simulink subsystem "robot_model_7dof_ref_subsys"  (R2022b)
settings: Solver=VariableStepAuto  StartTime=0.0  StopTime=10.0  RelTol=1e-3
undefined symbols (not defined in the file): param_robot, param_traj, q_0
settings Model: Creator=emu  LastModifiedBy=rslstudent
settings OptimizationCC: ReuseModelBlockBuffer=on

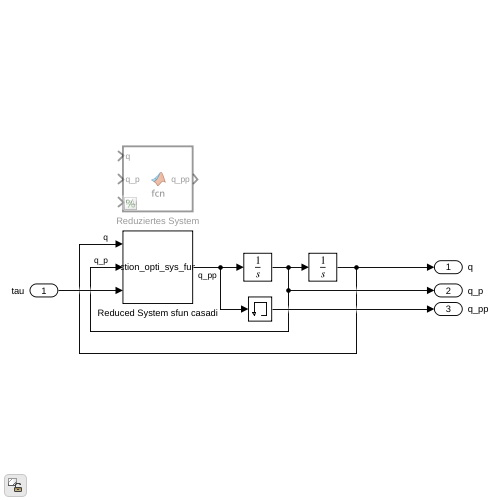
[thumbnail: Simulink's stored preview of the top-level diagram]
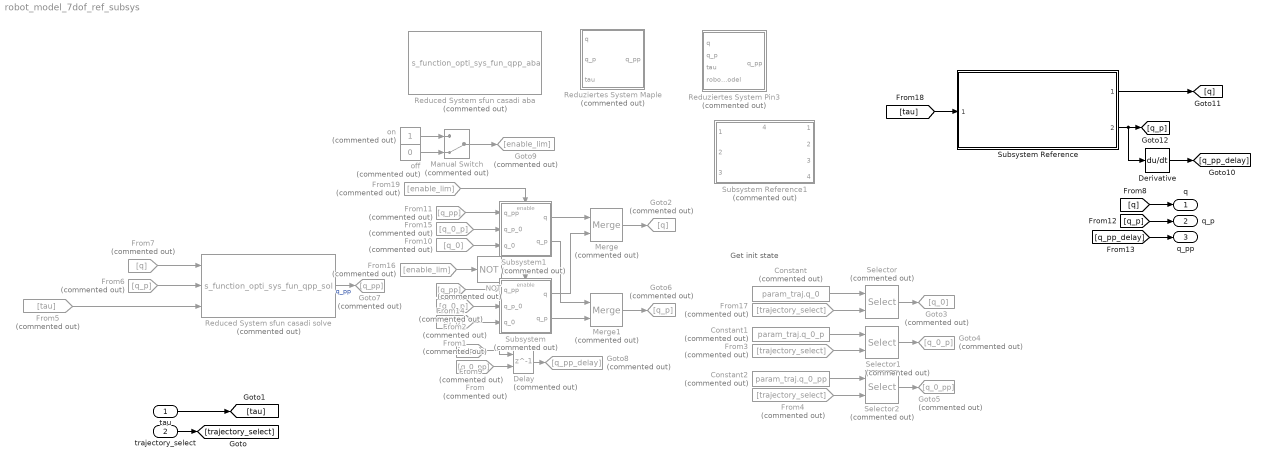
== system robot_model_7dof_ref_subsys ==
  note: Get init state
  tau : Inport
  trajectory_select : Inport  Port=2
  Constant : Constant  Commented=on  Value=param_traj.q_0
  Constant1 : Constant  Commented=on  Value=param_traj.q_0_p
  Constant2 : Constant  Commented=on  Value=param_traj.q_0_pp
  Delay : Delay  Commented=on  DelayLength=1  InitialConditionSource=Input port
      settings: InputPortMap=u0,p4
  Derivative : Derivative
  From : From  Commented=on  GotoTag=q_0_pp
  From1 : From  Commented=on  GotoTag=q_0
  From10 : From  Commented=on  GotoTag=q_0
  From11 : From  Commented=on  GotoTag=q_pp
  From14 : From  Commented=on  GotoTag=q_pp
  From15 : From  Commented=on  GotoTag=q_0_p
  From16 : From  Commented=on  GotoTag=enable_lim
  From17 : From  Commented=on  GotoTag=trajectory_select
  From19 : From  Commented=on  GotoTag=enable_lim
  From2 : From  Commented=on  GotoTag=q_0_p
  From3 : From  Commented=on  GotoTag=trajectory_select
  From4 : From  Commented=on  GotoTag=trajectory_select
  From5 : From  Commented=on  GotoTag=tau
  From6 : From  Commented=on  GotoTag=q_p
  From7 : From  Commented=on  GotoTag=q
  From9 : From  Commented=on  GotoTag=q_pp
  Goto2 : Goto  Commented=on  GotoTag=q
  Goto3 : Goto  Commented=on  GotoTag=q_0
  Goto4 : Goto  Commented=on  GotoTag=q_0_p
  Goto5 : Goto  Commented=on  GotoTag=q_0_pp
  Goto6 : Goto  Commented=on  GotoTag=q_p
  Goto7 : Goto  Commented=on  GotoTag=q_pp
  Goto8 : Goto  Commented=on  GotoTag=q_pp_delay
  Goto9 : Goto  Commented=on  GotoTag=enable_lim
  Manual Switch : ManualSwitch  Commented=on  CurrentSetting=0
  Merge : Merge  Commented=on
  Merge1 : Merge  Commented=on
  NOT : Logic  Commented=on  Operator=NOT  IconShape=distinctive  AllPortsSameDT=off  OutDataTypeStr=boolean
  Reduced System sfun casadi aba : S-Function  Commented=on  FunctionName=s_function_opti_sys_fun_qpp_aba  SFunctionModules='sys_fun_qpp_aba'  SFunctionDeploymentMode=off  EnableBusSupport=off
  Reduced System sfun casadi solve : S-Function  Commented=on  FunctionName=s_function_opti_sys_fun_qpp_sol  SFunctionModules='sys_fun_qpp_sol'  SFunctionDeploymentMode=off  EnableBusSupport=off
  Reduziertes System Maple : MATLAB Function  Commented=on
  Reduziertes System Pin3 : MATLAB Function  Commented=on
  Selector : Selector  Commented=on  NumberOfDimensions=2  InputPortWidth=3  IndexOptions=Index vector (dialog),Index vector (port)  Indices=1:param_robot.n_DOF,1  OutputSizes=1,1
  Selector1 : Selector  Commented=on  NumberOfDimensions=2  InputPortWidth=3  IndexOptions=Index vector (dialog),Index vector (port)  Indices=1:param_robot.n_DOF,1  OutputSizes=1,1
  Selector2 : Selector  Commented=on  NumberOfDimensions=2  InputPortWidth=3  IndexOptions=Index vector (dialog),Index vector (port)  Indices=1:param_robot.n_DOF,1  OutputSizes=1,1
  Subsystem : Subsystem  Commented=on
  Subsystem Reference : Subsystem  ReferencedSubsystem=franka_fr3_no_hand_simscape_model_refsys
  Subsystem Reference1 : Subsystem  Commented=on  ReferencedSubsystem=limit_joint_coordinates_ref_subsys
      settings: PortSchema="{\"entries\":[{\"content\":{\"sides\":[{\"content\":{\"connectorIds\":[\"In1\",\"In2\",\"In3\"]},\"type\":\"ConnectorPlacement.EquallySpacedRectSide\",\"uuid\":\"c83c87ef-f061-4ba1-866a-9dee58807a3f\"},{\"content\":{\"connectorIds\":[\"Out1\",\"Out2\",\"Out3\",\"Out4\"],\"side\":\"RIGHT\"},\"type\":\"ConnectorPlacement.EquallySpacedRectSide\",\"uuid\":\"387cc6c9-8217-4e2c-af30-f5a1ca09c27e\"},{\"content\":{\"connectorIds\":[\"In4\"],\"side\":\"TOP\"},\"type\":\"ConnectorPlacement.EquallySpacedRectSide\",\"uuid\":\"e929a290-99c7-445c-910f-8eb13519bf88\"}]},\"type\":\"ConnectorPlacement.EquallySpacedConnector\",\"uuid\":\"10c7422a-0646-4362-bf57-e7ffff3efdcc\"}],\"packageUris\":[\"http://schema.mathworks.com/mf0/Connector/R2020b\"],\"version\":\"1.0\"}"
  Subsystem1 : Subsystem  Commented=on
  off : Constant  Commented=on  Value=0
  on : Constant  Commented=on
  q : Outport
  q_p : Outport  Port=2
  q_pp : Outport  Port=3
  wires:
  Constant/1 -> Selector/1
  trajectory_select/1 -> [trajectory_select]
  Constant1/1 -> Selector1/1
  Constant2/1 -> Selector2/1
  Selector/1 -> Goto3/1
  Selector1/1 -> Goto4/1
  Selector2/1 -> Goto5/1
  From17/1 -> Selector/2
  From4/1 -> Selector2/2
  From3/1 -> Selector1/2
  [tau] -> Subsystem Reference/1
  Subsystem Reference/2 -> [q_p], Derivative/1
  Derivative/1 -> [q_pp_delay]
  From5/1 -> Reduced System sfun casadi solve/3
  tau/1 -> [tau]
  Subsystem Reference/1 -> [q]
  From6/1 -> Reduced System sfun casadi solve/2
  From7/1 -> Reduced System sfun casadi solve/1
  [q_pp_delay] -> q_pp/1
  [q_p] -> q_p/1
  [q] -> q/1
  off/1 -> Manual Switch/2
  on/1 -> Manual Switch/1
  Manual Switch/1 -> Goto9/1
  From14/1 -> Subsystem/1(q_pp)
  Reduced System sfun casadi solve/1 -> Goto7/1  "q_pp"
  Delay/1 -> Goto8/1
  From/1 -> Delay/2
  From2/1 -> Subsystem/2(q_p_0)
  From1/1 -> Subsystem/3(q_0)
  From9/1 -> Delay/1
  From10/1 -> Subsystem1/3(q_0)
  From15/1 -> Subsystem1/2(q_p_0)
  From11/1 -> Subsystem1/1(q_pp)
  NOT/1 -> Subsystem/Enable
  From16/1 -> NOT/1
  From19/1 -> Subsystem1/Enable
  Subsystem1/1(q) -> Merge/1
  Subsystem/1(q) -> Merge/2
  Subsystem1/2(q_p) -> Merge1/1
  Subsystem/2(q_p) -> Merge1/2
  Merge/1 -> Goto2/1
  Merge1/1 -> Goto6/1

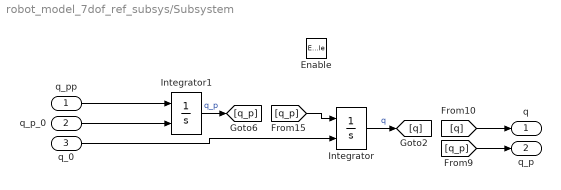
== system robot_model_7dof_ref_subsys/Subsystem ==
  q_pp : Inport
  q_p_0 : Inport  Port=2
  q_0 : Inport  Port=3
  Enable : EnablePort
  Integrator : Integrator  InitialConditionSource=external  InitialCondition=q_0  UpperSaturationLimit=param_robot.q_limit_upper  LowerSaturationLimit=param_robot.q_limit_lower
  Integrator1 : Integrator  InitialConditionSource=external  InitialCondition=param_robot.q_0_p_ref  UpperSaturationLimit=param_robot.q_p_limit_upper  LowerSaturationLimit=param_robot.q_p_limit_lower
  q : Outport
  q_p : Outport  Port=2
  wires:
  [q_p] -> q_p/1
  [q] -> q/1
  q_p_0/1 -> Integrator1/2
  q_0/1 -> Integrator/2
  Integrator1/1 -> [q_p]  "q_p"
  q_pp/1 -> Integrator1/1
  Integrator/1 -> [q]  "q"
  [q_p] -> Integrator/1

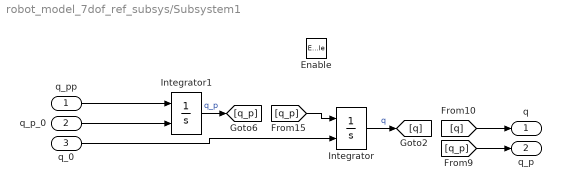
== system robot_model_7dof_ref_subsys/Subsystem1 ==
  q_pp : Inport
  q_p_0 : Inport  Port=2
  q_0 : Inport  Port=3
  Enable : EnablePort
  Integrator : Integrator  InitialConditionSource=external  InitialCondition=q_0  LimitOutput=on  UpperSaturationLimit=param_robot.q_limit_upper  LowerSaturationLimit=param_robot.q_limit_lower
  Integrator1 : Integrator  InitialConditionSource=external  InitialCondition=param_robot.q_0_p_ref  LimitOutput=on  UpperSaturationLimit=param_robot.q_p_limit_upper  LowerSaturationLimit=param_robot.q_p_limit_lower
  q : Outport
  q_p : Outport  Port=2
  wires:
  [q_p] -> Integrator/1
  Integrator/1 -> [q]  "q"
  q_pp/1 -> Integrator1/1
  Integrator1/1 -> [q_p]  "q_p"
  q_0/1 -> Integrator/2
  q_p_0/1 -> Integrator1/2
  [q] -> q/1
  [q_p] -> q_p/1

== matlab function robot_model_7dof_ref_subsys/Reduziertes System Maple ==
  data: q input; q_p input; tau input; q_pp output; param_robot parameter
function q_pp =fcn(q, q_p,tau, param_robot)

M=inertia_matrix(q,param_robot);                          % rigid body inertia matrix
C=coriolis_matrix(q,q_p,param_robot);                     % coriolis matrix
g=gravitational_forces(q,param_robot);                    % gravitational forces

q_pp = M\(tau - C*q_p - g);

% q_pp = M\(tau-C*q_p-g - 0.5*diag(ones(7,1))*q_p(3:9)); % mit Reibung

== matlab function robot_model_7dof_ref_subsys/Reduziertes System Pin3 ==
  data: q input; q_p input; tau input; robot_model input Bus: robot_model; q_pp output
function q_pp =fcn(q, q_p, tau, robot_model)
M = robot_model.M;
C_rnea = robot_model.C_rnea;

q_pp = M\(tau - C_rnea);
